simulink model "distance_measure"  (R2018b)
settings: Solver=FixedStepDiscrete  StartTime=0.0  StopTime=inf  FixedStep=1/200  RelTol=1e-3
values from neighbouring files (symbols this model uses):
  conf = Configuration    [config.m]
libraries: car_lib x1, sldrtlib x1
settings Model: Creator=petrb  LastModifiedBy=Lenovo
settings SolverCC: PositivePriorityOrder=on
settings OptimizationCC: PassReuseOutputArgsAs=Individual arguments  MaxStackSize=64
settings DebuggingCC: ParameterTunabilityLossMsg=error  LibraryContextMissingDiagnostic=none
settings HardwareCC: ProdBitPerPointer=32  ProdBitPerSizeT=32  ProdBitPerPtrDiffT=32  ProdLargestAtomicInteger=Long  ProdLargestAtomicFloat=Double  ProdWordSize=32  ProdHWDeviceType=ARM Compatible->ARM Cortex
settings SFSimCC: SimUseLocalCustomCode=off  MATLABDynamicMemAlloc=off
settings RTWCC: SystemTargetFile=ert.tlc  HardwareBoard=BeagleBone Blue  TLCOptions="-aInlineSetEventsForThisBaseRateFcn=TLC_FALSE -aSuppressMultiTaskScheduler=TLC_FALSE  -aRateBasedStepFcn=0"  TemplateMakefile=ert_default_tmf  RTWUseLocalCustomCode=off  RTWUseSimCustomCode=on  Toolchain=GNU GCC BeagleBone Blue  IncludeHyperlinkInReport=on
settings CodeAppCC: ForceParamTrailComments=on  IgnoreCustomStorageClasses=off  OperatorAnnotations=on  SimulinkDataObjDesc=on  SFDataObjDesc=on  InsertBlockDesc=on
settings ERTTargetCC: SupportNonInlinedSFcns=on  SupportVariableSizeSignals=on

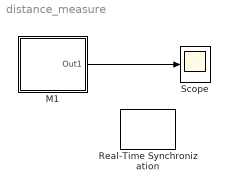
== system distance_measure ==
  M1 : Subsystem
  Real-Time Synchronization : sldrtlib/Real-Time Synchronization  SampleTime=conf.CommSampleTime  MaxMissedTicks=40402  ShowMissedTicks=off  YieldWhenWaiting=on
  Scope : Scope
  wires:
  M1/1(Out1) -> Scope/1

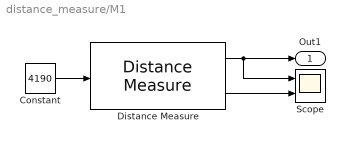
== system distance_measure/M1 ==
  Constant : Constant  Value=4190
  Distance Measure : car_lib/Distance Measure
  Scope : Scope  NumInputPorts=2
  Out1 : Outport
  wires:
  Distance Measure/1 -> Out1/1, Scope/1
  Constant/1 -> Distance Measure/1
  Distance Measure/2 -> Scope/2
